simulink model "sfcndemo_ada_multi_port"  (Simulink 6.0)
settings: Solver=FixedStepDiscrete  StartTime=0.0  StopTime=inf  RelTol=1e-3
settings Model: Creator=The MathWorks Inc.  LastModifiedBy=batserve  ExtModeAutoUpdateStatusClock=off
settings DataIOCC: SaveOutput=off  SaveTime=off
settings OptimizationCC: BlockReduction=off  BooleanDataType=off
settings DebuggingCC: ConsistencyChecking=error  ArrayBoundsChecking=error  CheckExecutionContextPreStartOutputMsg=on  CheckExecutionContextRuntimeOutputMsg=on  SolverPrmCheckMsg=none
settings HardwareCC: TargetUnknown=on

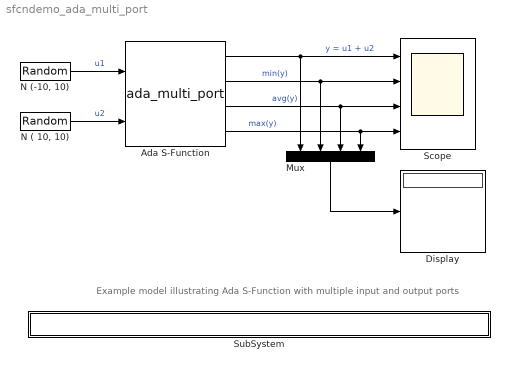
== system sfcndemo_ada_multi_port ==
  note: Example model illustrating Ada S-Function with multiple input and output ports
  Ada S-Function : S-Function  FunctionName=ada_multi_port  Parameters='++'
  Display : Display
  Mux : Mux  Orientation=down
  "N ( 10, 10)" : RandomNumber  Mean=10  Variance=10  Seed=1  SampleTime=0
  "N (-10, 10)" : RandomNumber  Mean=-10  Variance=10  SampleTime=0
  Scope : Scope  NumInputPorts=4
      settings: TimeRange=1000  YMin=-20~-20~-0.5~-20  YMax=20~20~0.5~20  DataFormat=Structure
  SubSystem : Subsystem  PropExecContextAcrossSSBoundary=on
      settings: OpenFcn=evalin('base','edit(fullfile(matlabroot,''simulink'',''ada'',''examples'',''multi_port'',''multi_port.adb''))')
      mask Display: disp('matlabroot\simulink\ada\examples\multi_port\multi_port.adb');
  wires:
  "N ( 10, 10)"/1 -> Ada S-Function/2  "u2"
  "N (-10, 10)"/1 -> Ada S-Function/1  "u1"
  Ada S-Function/1 -> Scope/1, Mux/1  "y = u1 + u2"
  Ada S-Function/2 -> Scope/2, Mux/2  "min(y)"
  Ada S-Function/3 -> Scope/3, Mux/3  "avg(y)"
  Ada S-Function/4 -> Scope/4, Mux/4  "max(y)"
  Mux/1 -> Display/1

== system sfcndemo_ada_multi_port/SubSystem ==
